simulink library "springFunc_block"  (R2019a)
settings: Solver=VariableStepAuto  StartTime=0.0  StopTime=10.0  RelTol=1e-3
settings Model: Creator=agmotes  LastModifiedBy=agmotes

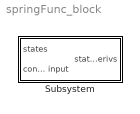
== system springFunc_block ==
  Subsystem : Subsystem  mask{c1=0, c2=0, c3=0}
      mask prompts: c1 "Mass"; c2 "Spring Constant"; c3 "Damping Constant"

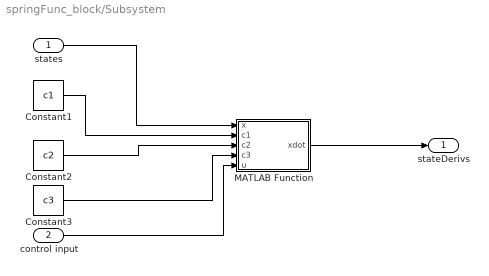
== system springFunc_block/Subsystem ==
  states : Inport
  control input : Inport  Port=2
  Constant1 : Constant  Value=c1
  Constant2 : Constant  Value=c2
  Constant3 : Constant  Value=c3
  MATLAB Function : MATLAB Function  TreatAsAtomicUnit=on
  stateDerivs : Outport
  wires:
  states/1 -> MATLAB Function/1(x)
  MATLAB Function/1(xdot) -> stateDerivs/1
  Constant1/1 -> MATLAB Function/2(c1)
  Constant2/1 -> MATLAB Function/3(c2)
  Constant3/1 -> MATLAB Function/4(c3)
  control input/1 -> MATLAB Function/5(u)

== matlab function springFunc_block/Subsystem/MATLAB Function ==
  data: x input; xdot output; c1 input; c2 input; c3 input; u input
function xdot  = springFunc(x,c1,c2,c3,u)
    
    xdot = zeros(1,2);

    m = c1;
    k = c2;
    b = c3;

	xdot(1) = x(2);
	xdot(2) = u-(b*x(2) + k*x(1))/m;

	%xdot = xdot';
